simulink library "Plants"  (R2023b)
settings: Solver=VariableStepAuto  StartTime=0.0  StopTime=10.0  RelTol=1e-3
PreLoadFcn:
  | PlantsInit;
values from neighbouring files (symbols this model uses):
  blockschaltbildKoeffizienten = [0.0637851 -0.0232653 189.219 -0.207233 18.8808 -0.809018 -0.228862 ]    [PlantsInit.m]
undefined symbols (not defined in the file or in its folder): motorMitSchwungmasseStateSpace
libraries: simulink x5, models x1
settings Model: Creator=Alex  LastModifiedBy=Alex

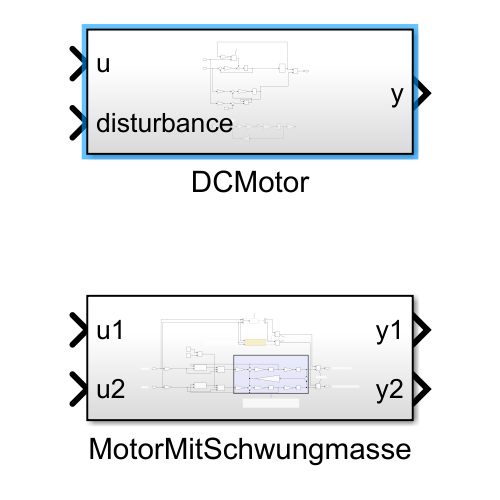
[thumbnail: Simulink's stored preview of the top-level diagram]
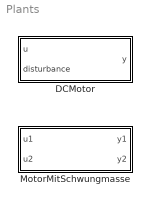
== system Plants ==
  DCMotor : Subsystem
  MotorMitSchwungmasse : Subsystem  InitFcn=|
      | if exist('MotorMitSchwungmasse', 'var')
      |     disp('MotorMitSchwungmasse exists!');
      | else
      |     PlantsInit;
      | end

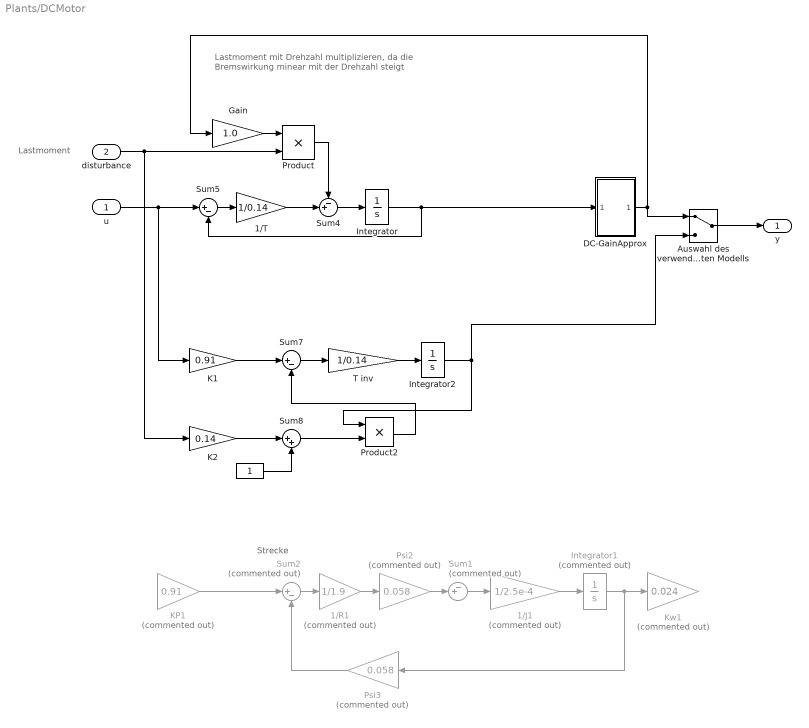
== system Plants/DCMotor ==
  note: Lastmoment mit Drehzahl multiplizieren,
      | da die Bremswirkung minear mit der Drehzahl steigt
  note: Lastmoment
  note: Strecke
  u : Inport
  disturbance : Inport  Port=2
  " " : Constant
  1/J1 : Gain  Commented=on  Gain=1/2.5e-4  SaturateOnIntegerOverflow=on  OutDataTypeStr=Inherit: Same as input  ParamDataTypeStr=Inherit: Same as input
  1/R1 : Gain  Commented=on  Gain=1/1.9  SaturateOnIntegerOverflow=on  OutDataTypeStr=Inherit: Same as input  ParamDataTypeStr=Inherit: Same as input
  1/T : Gain  Gain=1/0.14  SaturateOnIntegerOverflow=on  OutDataTypeStr=Inherit: Same as input  ParamDataTypeStr=Inherit: Same as input
  Auswahl des verwendeten Modells : ManualSwitch
  DC-GainApprox : Subsystem
  Gain : Gain  Gain=1.0
  Integrator : Integrator
  Integrator1 : Integrator  Commented=on
  Integrator2 : Integrator
  K1 : Gain  Gain=0.91
  K2 : Gain  Gain=0.14
  KP1 : Gain  Commented=on  Gain=0.91  SaturateOnIntegerOverflow=on  OutDataTypeStr=Inherit: Same as input  ParamDataTypeStr=Inherit: Same as input
  Kw1 : Gain  Commented=on  Gain=0.024  SaturateOnIntegerOverflow=on  OutDataTypeStr=Inherit: Same as input  ParamDataTypeStr=Inherit: Same as input
  Product : Product
  Product2 : Product
  Psi2 : Gain  Commented=on  Gain=0.058  SaturateOnIntegerOverflow=on  OutDataTypeStr=Inherit: Same as input  ParamDataTypeStr=Inherit: Same as input
  Psi3 : Gain  Commented=on  Gain=0.058  SaturateOnIntegerOverflow=on  OutDataTypeStr=Inherit: Same as input  ParamDataTypeStr=Inherit: Same as input
  Sum1 : Sum  Commented=on  Inputs=-+|  InputSameDT=on  SaturateOnIntegerOverflow=on  OutDataTypeStr=Inherit: Same as first input
  Sum2 : Sum  Commented=on  Inputs=|+-  InputSameDT=on  SaturateOnIntegerOverflow=on  OutDataTypeStr=Inherit: Same as first input
  Sum4 : Sum  Inputs=-+|  InputSameDT=on  SaturateOnIntegerOverflow=on  OutDataTypeStr=Inherit: Same as first input
  Sum5 : Sum  Inputs=|+-  InputSameDT=on  SaturateOnIntegerOverflow=on  OutDataTypeStr=Inherit: Same as first input
  Sum7 : Sum  Inputs=|+-  InputSameDT=on  SaturateOnIntegerOverflow=on  OutDataTypeStr=Inherit: Same as first input
  Sum8 : Sum  Inputs=|++  InputSameDT=on  SaturateOnIntegerOverflow=on  OutDataTypeStr=Inherit: Same as first input
  T inv : Gain  Gain=1/0.14
  y : Outport
  wires:
  u/1 -> K1/1, Sum5/1
  Gain/1 -> Product/1
  disturbance/1 -> Product/2, K2/1
  KP1/1 -> Sum2/1
  Integrator1/1 -> Psi3/1, Kw1/1
  1/J1/1 -> Integrator1/1
  1/R1/1 -> Psi2/1
  Sum2/1 -> 1/R1/1
  Psi3/1 -> Sum2/2
  Sum1/1 -> 1/J1/1
  Psi2/1 -> Sum1/2
  Sum5/1 -> 1/T/1
  1/T/1 -> Sum4/2
  Sum4/1 -> Integrator/1
  Product/1 -> Sum4/1
  Integrator/1 -> DC-GainApprox/1(In1), Sum5/2
  Auswahl des verwendeten Modells/1 -> y/1
  " "/1 -> Sum8/2
  K2/1 -> Sum8/1
  K1/1 -> Sum7/1
  Sum8/1 -> Product2/2
  Integrator2/1 -> Auswahl des verwendeten Modells/2, Product2/1
  Product2/1 -> Sum7/2
  T inv/1 -> Integrator2/1
  Sum7/1 -> T inv/1
  DC-GainApprox/1(Out1) -> Gain/1, Auswahl des verwendeten Modells/1

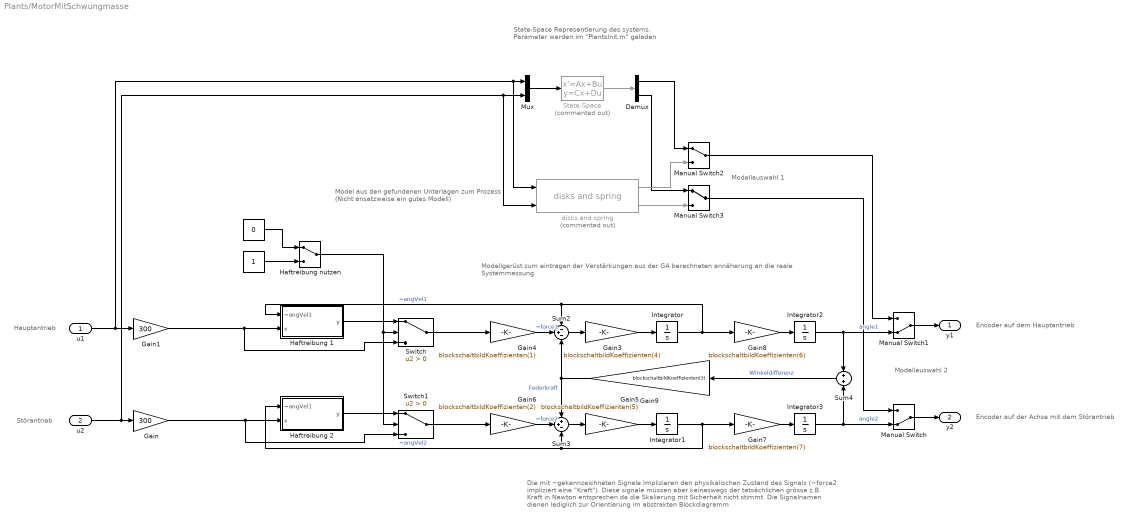
== system Plants/MotorMitSchwungmasse ==
  note: Encoder auf dem Hauptantrieb
  note: Störantrieb
  note: Hauptantrieb
  note: Modellauswahl 1
  note: State-Space Representierung des systems.
      | Parameter werden im "PlantsInit.m" geladen
  note: Die mit ~gekennzeichneten Signale Implizieren den physikalischen Zustand des Signals (~force2 impliziert eine "Kraft"). Diese signale müssen aber keineswegs der tatsächlichen grösse z.B. Kraft in Newton entsprechen da die Skalierung mit Sicherheit nicht stimmt.
      |
      | Die Signalnamen dienen lediglich zur Orientierung im abstrakten Blockdiagramm
  note: Modellgerüst zum eintragen der Verstärkungen aus der GA berechneten annäherung
      | an die reale Systemmessung
  note: Model aus den gefundenen Unterlagen zum Prozess
      | (Nicht ansatzweise ein gutes Modell)
  note: Modellauswahl 2
  note: Encoder auf der Achse mit dem Störantrieb
  u1 : Inport
  u2 : Inport  Port=2
  " " : Constant
  "   " : Constant  Value=0
  Demux : Demux  Outputs=2
  Gain : Gain  Gain=300
  Gain1 : Gain  Gain=300
  Gain3 : Gain  Gain=blockschaltbildKoeffizienten(4)
  Gain4 : Gain  Gain=blockschaltbildKoeffizienten(1)
  Gain5 : Gain  Gain=blockschaltbildKoeffizienten(5)
  Gain6 : Gain  Gain=blockschaltbildKoeffizienten(2)
  Gain7 : Gain  Gain=blockschaltbildKoeffizienten(7)
  Gain8 : Gain  Gain=blockschaltbildKoeffizienten(6)
  Gain9 : Gain  Gain=blockschaltbildKoeffizienten(3)
  Haftreibung 1 : Subsystem
  Haftreibung 2 : Subsystem
  Haftreibung nutzen : ManualSwitch
  Integrator{,1..3} (4 alike) : Integrator
  Manual Switch : ManualSwitch  CurrentSetting=0
  Manual Switch1 : ManualSwitch  CurrentSetting=0
  Manual Switch2 : ManualSwitch
  Manual Switch3 : ManualSwitch
  Mux : Mux  Inputs=2
  State-Space : StateSpace  Commented=on  A=motorMitSchwungmasseStateSpace.A  B=motorMitSchwungmasseStateSpace.B  C=motorMitSchwungmasseStateSpace.C  D=motorMitSchwungmasseStateSpace.D  InitialCondition=0
  Sum2 : Sum  Inputs=-+-
  Sum3 : Sum  Inputs=++-
  Sum4 : Sum  Inputs=+|+
  Switch : Switch  Criteria=u2 > Threshold  SaturateOnIntegerOverflow=off  InputSameDT=off
  Switch1 : Switch  Criteria=u2 > Threshold  SaturateOnIntegerOverflow=off  InputSameDT=off
  disks and spring : models/disks and spring  Commented=on  theta1=theta1  d1=d1  theta2=theta2  d2=d2  c=c  d=d  kt1=kt1  kt2=kt2
  y1 : Outport
  y2 : Outport  Port=2
  wires:
  Mux/1 -> State-Space/1
  Manual Switch2/1 -> Manual Switch1/1
  Manual Switch3/1 -> Manual Switch/1
  State-Space/1 -> Demux/1
  Sum2/1 -> Gain3/1
  Gain3/1 -> Integrator/1
  Gain4/1 -> Sum2/2  "~force1"
  Integrator/1 -> Haftreibung 1/1(~angVel1), Sum2/1, Gain8/1  "~angVel1"
  Integrator2/1 -> Sum4/1, Manual Switch1/2  "angle1"
  Integrator1/1 -> Sum3/3, Haftreibung 2/1(~angVel1), Gain7/1  "~angVel2"
  Gain5/1 -> Integrator1/1
  Sum3/1 -> Gain5/1
  Integrator3/1 -> Sum4/2, Manual Switch/2  "angle2"
  Gain7/1 -> Integrator3/1
  Gain8/1 -> Integrator2/1
  Gain9/1 -> Sum3/1, Sum2/3  "Federkraft"
  Gain6/1 -> Sum3/2  "~force2"
  Sum4/1 -> Gain9/1  "Winkeldifferenz"
  Manual Switch/1 -> y2/1
  Manual Switch1/1 -> y1/1
  u2/1 -> Gain/1, disks and spring/2, Mux/2
  Haftreibung 2/1(y) -> Switch1/1
  Demux/1 -> Manual Switch2/1
  Demux/2 -> Manual Switch3/1
  disks and spring/1 -> Manual Switch2/2
  disks and spring/2 -> Manual Switch3/2
  u1/1 -> disks and spring/1, Mux/1, Gain1/1
  Gain/1 -> Switch1/3, Haftreibung 2/2(x)
  Gain1/1 -> Switch/3, Haftreibung 1/2(x)
  Haftreibung 1/1(y) -> Switch/1
  Switch/1 -> Gain4/1
  Switch1/1 -> Gain6/1
  " "/1 -> Haftreibung nutzen/2
  "   "/1 -> Haftreibung nutzen/1
  Haftreibung nutzen/1 -> Switch1/2, Switch/2

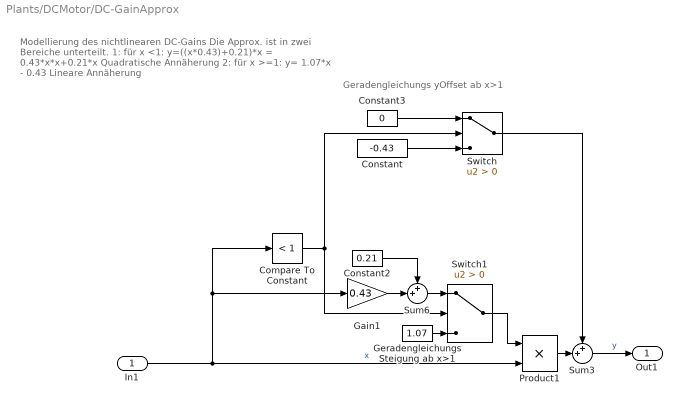
== system Plants/DCMotor/DC-GainApprox ==
  note: Geradengleichungs yOffset ab x>1
  note: Modellierung des nichtlinearen DC-Gains
      | Die Approx. ist in zwei Bereiche unterteilt.
      | 1: für x <1: y=((x*0.43)+0.21)*x = 0.43*x*x+0.21*x     Quadratische Annäherung
      |
      | 2: für x >=1: y= 1.07*x - 0.43
      | Lineare Annäherung
  In1 : Inport
  Compare To Constant : simulink/Logic and Bit Operations/Compare To Constant  relop=<  const=1  OutDataTypeStr=boolean
  Constant : Constant  Value=-0.43
  Constant2 : Constant  Value=0.21
  Constant3 : Constant  Value=0
  Gain1 : Gain  Gain=0.43
  Geradengleichungs Steigung ab x>1 : Constant  Value=1.07
  Product1 : Product
  Sum3 : Sum  Inputs=++|  InputSameDT=on  SaturateOnIntegerOverflow=on  OutDataTypeStr=Inherit: Same as first input
  Sum6 : Sum  Inputs=++|  InputSameDT=on  SaturateOnIntegerOverflow=on  OutDataTypeStr=Inherit: Same as first input
  Switch : Switch  Criteria=u2 > Threshold  SaturateOnIntegerOverflow=off  InputSameDT=off
  Switch1 : Switch  Criteria=u2 > Threshold  SaturateOnIntegerOverflow=off  InputSameDT=off
  Out1 : Outport
  wires:
  Constant/1 -> Switch/3
  Compare To Constant/1 -> Switch/2, Switch1/2
  Geradengleichungs Steigung ab x>1/1 -> Switch1/3
  Gain1/1 -> Sum6/2
  Product1/1 -> Sum3/2
  Sum6/1 -> Switch1/1
  Constant3/1 -> Switch/1
  Switch/1 -> Sum3/1
  Constant2/1 -> Sum6/1
  Switch1/1 -> Product1/1
  Sum3/1 -> Out1/1  "y"
  In1/1 -> Product1/2, Gain1/1, Compare To Constant/1  "x"

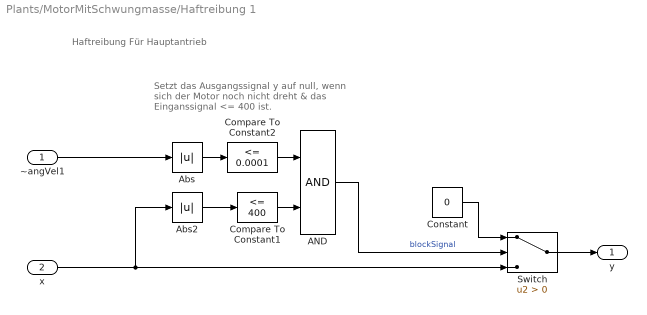
== system Plants/MotorMitSchwungmasse/Haftreibung 1 ==
  note: Haftreibung Für Hauptantrieb
  note: Setzt das Ausgangssignal y auf null,
      |    wenn sich der Motor noch nicht dreht &
      |    das Einganssignal <= 400 ist.
  ~angVel1 : Inport
  x : Inport  Port=2
  AND : Logic  IconShape=distinctive  AllPortsSameDT=off  OutDataTypeStr=boolean
  Abs : Abs  SaturateOnIntegerOverflow=off
  Abs2 : Abs  SaturateOnIntegerOverflow=off
  Compare To Constant1 : simulink/Logic and Bit Operations/Compare To Constant  relop=<=  const=400  OutDataTypeStr=boolean
  Compare To Constant2 : simulink/Logic and Bit Operations/Compare To Constant  relop=<=  const=0.0001  OutDataTypeStr=boolean
  Constant : Constant  Value=0
  Switch : Switch  Criteria=u2 > Threshold  SaturateOnIntegerOverflow=off  InputSameDT=off
  y : Outport
  wires:
  AND/1 -> Switch/2  "blockSignal"
  Compare To Constant2/1 -> AND/1
  x/1 -> Abs2/1, Switch/3
  Compare To Constant1/1 -> AND/2
  Abs2/1 -> Compare To Constant1/1
  Abs/1 -> Compare To Constant2/1
  Constant/1 -> Switch/1
  ~angVel1/1 -> Abs/1
  Switch/1 -> y/1

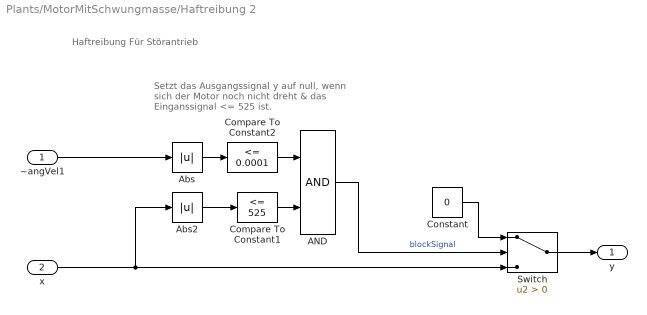
== system Plants/MotorMitSchwungmasse/Haftreibung 2 ==
  note: Haftreibung Für Störantrieb
  note: Setzt das Ausgangssignal y auf null,
      |    wenn sich der Motor noch nicht dreht &
      |    das Einganssignal <= 525 ist.
  ~angVel1 : Inport
  x : Inport  Port=2
  AND : Logic  IconShape=distinctive  AllPortsSameDT=off  OutDataTypeStr=boolean
  Abs : Abs  SaturateOnIntegerOverflow=off
  Abs2 : Abs  SaturateOnIntegerOverflow=off
  Compare To Constant1 : simulink/Logic and Bit Operations/Compare To Constant  relop=<=  const=525  OutDataTypeStr=boolean
  Compare To Constant2 : simulink/Logic and Bit Operations/Compare To Constant  relop=<=  const=0.0001  OutDataTypeStr=boolean
  Constant : Constant  Value=0
  Switch : Switch  Criteria=u2 > Threshold  SaturateOnIntegerOverflow=off  InputSameDT=off
  y : Outport
  wires:
  Compare To Constant1/1 -> AND/2
  Compare To Constant2/1 -> AND/1
  AND/1 -> Switch/2  "blockSignal"
  Abs2/1 -> Compare To Constant1/1
  ~angVel1/1 -> Abs/1
  Switch/1 -> y/1
  Constant/1 -> Switch/1
  x/1 -> Abs2/1, Switch/3
  Abs/1 -> Compare To Constant2/1
